simulink model "gm_fixed_point"  (R2022b)
settings: Solver=VariableStepAuto  StartTime=0.0  StopTime=1000.0  RelTol=1e-3
settings Model: Creator=Вячеслав  LastModifiedBy=Вячеслав
settings OptimizationCC: BlockReduction=off  ConditionallyExecuteInputs=off
settings DebuggingCC: InheritedTsInSrcMsg=none

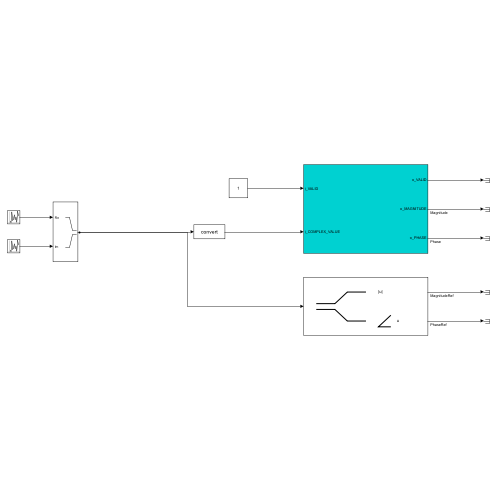
[thumbnail: Simulink's stored preview of the top-level diagram]
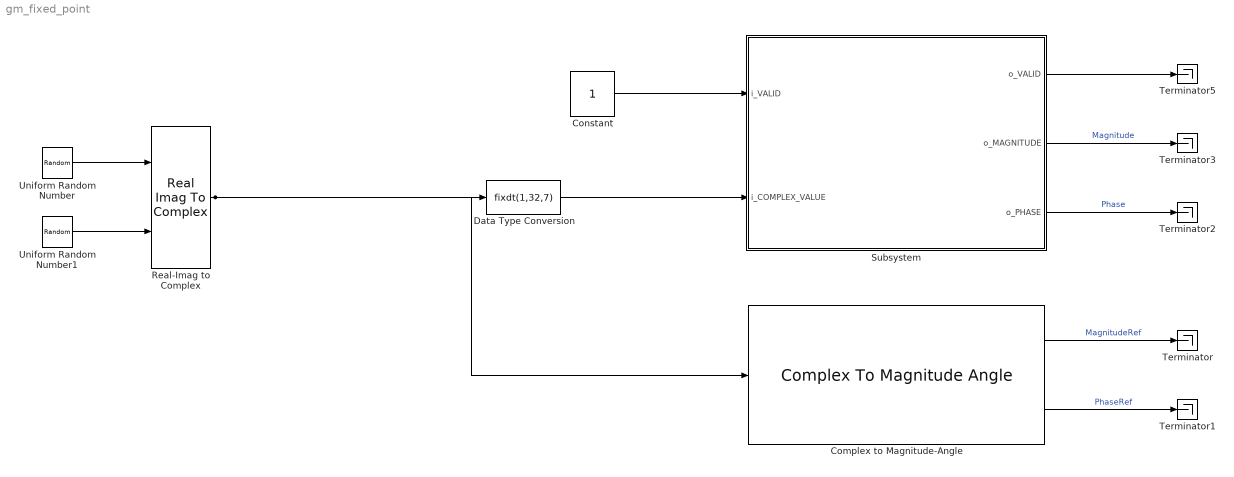
== system gm_fixed_point ==
  Complex to Magnitude-Angle : ComplexToMagnitudeAngle
  Constant : Constant  OutDataTypeStr=boolean  SampleTime=-1
  Data Type Conversion : DataTypeConversion  OutDataTypeStr=fixdt(1,32,7)  RndMeth=Round  SaturateOnIntegerOverflow=off
  Real-Imag to Complex : RealImagToComplex
  Subsystem : Subsystem
  Terminator{,1..3,5} (5 alike) : Terminator
  Uniform Random Number : UniformRandomNumber  Minimum=-2^(25-1)  Maximum=2^(25-1)-1/2^7  Seed=25  SampleTime=1
  Uniform Random Number1 : UniformRandomNumber  Minimum=-2^(25-1)  Maximum=2^(25-1)-1/2^7  Seed=26  SampleTime=1
  wires:
  Uniform Random Number1/1 -> Real-Imag to Complex/2
  Uniform Random Number/1 -> Real-Imag to Complex/1
  Real-Imag to Complex/1 -> Complex to Magnitude-Angle/1, Data Type Conversion/1
  Constant/1 -> Subsystem/1(i_VALID)
  Complex to Magnitude-Angle/1 -> Terminator/1  "MagnitudeRef"
  Complex to Magnitude-Angle/2 -> Terminator1/1  "PhaseRef"
  Subsystem/2(o_MAGNITUDE) -> Terminator3/1  "Magnitude"
  Subsystem/3(o_PHASE) -> Terminator2/1  "Phase"
  Subsystem/1(o_VALID) -> Terminator5/1
  Data Type Conversion/1 -> Subsystem/2(i_COMPLEX_VALUE)

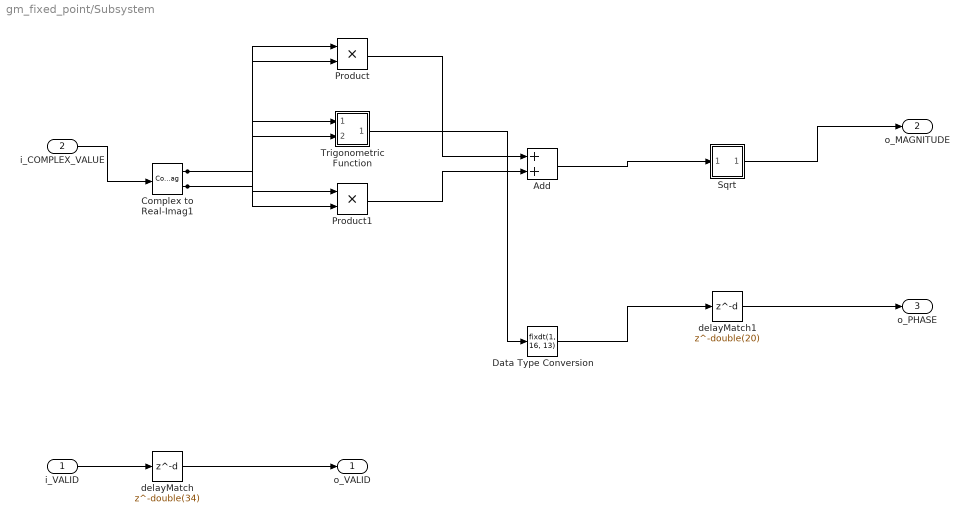
== system gm_fixed_point/Subsystem ==
  i_VALID : Inport  OutDataTypeStr=boolean  PortDimensions=1  SampleTime=1
  i_COMPLEX_VALUE : Inport  Port=2  OutDataTypeStr=fixdt(1, 32, 7)  PortDimensions=1  SampleTime=1  LockScale=on
      settings: SignalType=complex
  Add : Sum  AccumDataTypeStr=fixdt(1, 64, 14)  OutDataTypeStr=fixdt(1, 64, 14)  SampleTime=1
  Complex to Real-Imag1 : ComplexToRealImag  SampleTime=1
  Data Type Conversion : DataTypeConversion  OutDataTypeStr=fixdt(1, 16, 13)  RndMeth=Round  SampleTime=1  SaturateOnIntegerOverflow=off
  Product : Product  Inputs=**  OutDataTypeStr=fixdt(1, 64, 14)  SampleTime=1
  Product1 : Product  Inputs=**  OutDataTypeStr=fixdt(1, 64, 14)  SampleTime=1
  Sqrt : Subsystem
  Trigonometric Function : Subsystem
  delayMatch : Delay  DelayLength=double(34)  InitialCondition=0  SampleTime=1
  delayMatch1 : Delay  DelayLength=double(20)  InitialCondition=0  SampleTime=1
  o_VALID : Outport  OutDataTypeStr=boolean  SampleTime=1
  o_MAGNITUDE : Outport  Port=2  SampleTime=1
  o_PHASE : Outport  Port=3  SampleTime=1
  wires:
  delayMatch/1 -> o_VALID/1
  i_COMPLEX_VALUE/1 -> Complex to Real-Imag1/1
  Add/1 -> Sqrt/1(In1)
  Complex to Real-Imag1/1 -> Product/2, Product/1, Trigonometric Function/2(In2)
  Complex to Real-Imag1/2 -> Product1/2, Product1/1, Trigonometric Function/1(In1)
  delayMatch1/1 -> o_PHASE/1
  Product/1 -> Add/1
  Product1/1 -> Add/2
  Sqrt/1(Out1) -> o_MAGNITUDE/1
  Trigonometric Function/1(Out1) -> Data Type Conversion/1
  i_VALID/1 -> delayMatch/1
  Data Type Conversion/1 -> delayMatch1/1

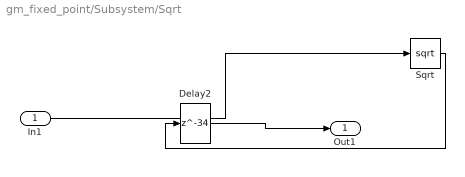
== system gm_fixed_point/Subsystem/Sqrt ==
  In1 : Inport
  Delay2 : Delay  DelayLength=34
  Sqrt : Sqrt  OutDataTypeStr=fixdt(1,33,7)
  Out1 : Outport
  wires:
  In1/1 -> Sqrt/1
  Sqrt/1 -> Delay2/1
  Delay2/1 -> Out1/1

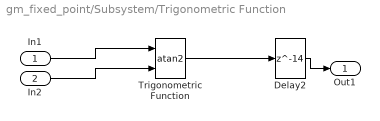
== system gm_fixed_point/Subsystem/Trigonometric Function ==
  In1 : Inport
  In2 : Inport  Port=2
  Delay2 : Delay  DelayLength=14
  Trigonometric Function : Trigonometry  Operator=atan2  ApproximationMethod=CORDIC
  Out1 : Outport
  wires:
  In1/1 -> Trigonometric Function/1
  In2/1 -> Trigonometric Function/2
  Trigonometric Function/1 -> Delay2/1
  Delay2/1 -> Out1/1
